simulink model "AS_H_Balanced_Load_7Bus"  (R2021a)
settings: Solver=ode45  StartTime=0.0  StopTime=1  RelTol=1e-3  EnableMultiTasking=on
undefined symbols (not defined in the file): D1, Delta
libraries: simulink_extras x12, spsDCVoltageSourceLib x12, spsDiodeLib x12, spsSeriesRLCBranchLib x12, spsGroundLib x10, spsRMSLib x8, dspstat3 x7, spsThreePhaseTransformerTwoWindingsLib x7, spsBreakerLib x7, spsThreePhaseSeriesRLCBranchLib x6, spsThreePhaseParallelRLCLoadLib x5, eePMU x4
(part 2 of 2)

== system AS_H_Balanced_Load_7Bus/HIF/HIF Fault/HIF4 ==
  DC Voltage Source : spsDCVoltageSourceLib/DC Voltage Source  Amplitude=2000  Measurements=None
  DC Voltage Source1 : spsDCVoltageSourceLib/DC Voltage Source  Amplitude=3000  Measurements=None
  Diode : spsDiodeLib/Diode  Ron=0.001  Lon=0  Vf=0.8  IC=0  UseSnubber=off  Rs=500  Cs=250e-9  Measurements=on
  Diode1 : spsDiodeLib/Diode  Ron=0.001  Lon=0  Vf=0.8  IC=0  UseSnubber=off  Rs=500  Cs=250e-9  Measurements=on
  Series RLC Branch : spsSeriesRLCBranchLib/Series RLC Branch  LConnTagsString=__new0  RConnTagsString=__new0  BranchType=R  Resistance=560  Inductance=1e-3  SetiL0=off  InitialCurrent=0  Capacitance=1e-6  Setx0=off  InitialVoltage=0  Measurements=None
  Series RLC Branch1 : spsSeriesRLCBranchLib/Series RLC Branch  LConnTagsString=__new0  RConnTagsString=__new0  BranchType=R  Resistance=560  Inductance=1e-3  SetiL0=off  InitialCurrent=0  Capacitance=1e-6  Setx0=off  InitialVoltage=0  Measurements=None
  Terminator : Terminator
  Terminator1 : Terminator
  + : PMIOPort  Side=Left
  - : PMIOPort  Port=2  Side=Right
  wires:
  Diode/1 -> Terminator/1
  Diode1/1 -> Terminator1/1
  connections:
  Series RLC Branch1/RConn1 -- Diode/LConn1
  DC Voltage Source1/RConn1 -- Diode/RConn1
  DC Voltage Source1/LConn1 -- DC Voltage Source/RConn1 -- -/RConn1
  Series RLC Branch/RConn1 -- Diode1/RConn1
  Series RLC Branch/LConn1 -- Series RLC Branch1/LConn1 -- +/RConn1
  DC Voltage Source/LConn1 -- Diode1/LConn1

== system AS_H_Balanced_Load_7Bus/HIF/HIF Fault/HIF5 ==
  DC Voltage Source : spsDCVoltageSourceLib/DC Voltage Source  Amplitude=2100  Measurements=None
  DC Voltage Source1 : spsDCVoltageSourceLib/DC Voltage Source  Amplitude=3100  Measurements=None
  Diode : spsDiodeLib/Diode  Ron=0.001  Lon=0  Vf=0.8  IC=0  UseSnubber=off  Rs=500  Cs=250e-9  Measurements=on
  Diode1 : spsDiodeLib/Diode  Ron=0.001  Lon=0  Vf=0.8  IC=0  UseSnubber=off  Rs=500  Cs=250e-9  Measurements=on
  Series RLC Branch : spsSeriesRLCBranchLib/Series RLC Branch  LConnTagsString=__new0  RConnTagsString=__new0  BranchType=R  Resistance=580  Inductance=1e-3  SetiL0=off  InitialCurrent=0  Capacitance=1e-6  Setx0=off  InitialVoltage=0  Measurements=None
  Series RLC Branch1 : spsSeriesRLCBranchLib/Series RLC Branch  LConnTagsString=__new0  RConnTagsString=__new0  BranchType=R  Resistance=580  Inductance=1e-3  SetiL0=off  InitialCurrent=0  Capacitance=1e-6  Setx0=off  InitialVoltage=0  Measurements=None
  Terminator : Terminator
  Terminator1 : Terminator
  + : PMIOPort  Side=Left
  - : PMIOPort  Port=2  Side=Right
  wires:
  Diode/1 -> Terminator/1
  Diode1/1 -> Terminator1/1
  connections:
  Series RLC Branch1/RConn1 -- Diode/LConn1
  DC Voltage Source1/RConn1 -- Diode/RConn1
  DC Voltage Source1/LConn1 -- DC Voltage Source/RConn1 -- -/RConn1
  Series RLC Branch/RConn1 -- Diode1/RConn1
  Series RLC Branch/LConn1 -- Series RLC Branch1/LConn1 -- +/RConn1
  DC Voltage Source/LConn1 -- Diode1/LConn1

== system AS_H_Balanced_Load_7Bus/HIF/HIF Fault/HIF6 ==
  DC Voltage Source : spsDCVoltageSourceLib/DC Voltage Source  Amplitude=2200  Measurements=None
  DC Voltage Source1 : spsDCVoltageSourceLib/DC Voltage Source  Amplitude=3200  Measurements=None
  Diode : spsDiodeLib/Diode  Ron=0.001  Lon=0  Vf=0.8  IC=0  UseSnubber=off  Rs=500  Cs=250e-9  Measurements=on
  Diode1 : spsDiodeLib/Diode  Ron=0.001  Lon=0  Vf=0.8  IC=0  UseSnubber=off  Rs=500  Cs=250e-9  Measurements=on
  Series RLC Branch : spsSeriesRLCBranchLib/Series RLC Branch  LConnTagsString=__new0  RConnTagsString=__new0  BranchType=R  Resistance=600  Inductance=1e-3  SetiL0=off  InitialCurrent=0  Capacitance=1e-6  Setx0=off  InitialVoltage=0  Measurements=None
  Series RLC Branch1 : spsSeriesRLCBranchLib/Series RLC Branch  LConnTagsString=__new0  RConnTagsString=__new0  BranchType=R  Resistance=600  Inductance=1e-3  SetiL0=off  InitialCurrent=0  Capacitance=1e-6  Setx0=off  InitialVoltage=0  Measurements=None
  Terminator : Terminator
  Terminator1 : Terminator
  + : PMIOPort  Side=Left
  - : PMIOPort  Port=2  Side=Right
  wires:
  Diode/1 -> Terminator/1
  Diode1/1 -> Terminator1/1
  connections:
  Series RLC Branch1/RConn1 -- Diode/LConn1
  DC Voltage Source1/RConn1 -- Diode/RConn1
  DC Voltage Source1/LConn1 -- DC Voltage Source/RConn1 -- -/RConn1
  Series RLC Branch/RConn1 -- Diode1/RConn1
  Series RLC Branch/LConn1 -- Series RLC Branch1/LConn1 -- +/RConn1
  DC Voltage Source/LConn1 -- Diode1/LConn1

== matlab function AS_H_Balanced_Load_7Bus/Energy Detector 11kV/Negative & Zero ED /Energy 11 kV ==
  data: P input; Energy output; t input
function Energy= fcn(P,t)
Energy=P*t;
%#codegen

== matlab function AS_H_Balanced_Load_7Bus/Energy Detector 33kVSide1/Energy 33 kV ==
  data: P input; Energy output; t input
function Energy= fcn(P,t)
Energy=P*t;
%#codegen
